simulink model "point_cloud_fusion_node"  (R2021b)
settings: Solver=FixedStepAuto  StartTime=0.0  StopTime=10.0  RelTol=1e-3
model workspace (MAT data in the model file):
  SL_ROS_VariableLengthArrays_MaxSizes.CommonInfo.ArrayTruncateAction = 'EmitWarning'
  SL_ROS_VariableLengthArrays_MaxSizes.MsgTypeMap = containers.Map
  SL_ROS_VariableLengthArrays_MaxSizes.MsgTypeMap.serialization.keys = {'sensor_msgs/PointCloud2'}
  SL_ROS_VariableLengthArrays_MaxSizes.MsgTypeMap.serialization.values{1}(1).PropertyName = 'data'
  SL_ROS_VariableLengthArrays_MaxSizes.MsgTypeMap.serialization.values{1}(1).DataType = 'uint8'
  SL_ROS_VariableLengthArrays_MaxSizes.MsgTypeMap.serialization.values{1}(1).MaxLength = 55000
  SL_ROS_VariableLengthArrays_MaxSizes.MsgTypeMap.serialization.values{1}(2).PropertyName = 'fields'
  SL_ROS_VariableLengthArrays_MaxSizes.MsgTypeMap.serialization.values{1}(2).DataType = 'sensor_msgs/PointField'
  SL_ROS_VariableLengthArrays_MaxSizes.MsgTypeMap.serialization.values{1}(2).MaxLength = 16
  SL_ROS_VariableLengthArrays_MaxSizes.MsgTypeMap.serialization.uniformity = 0
  SL_ROS_VariableLengthArrays_MaxSizes.MsgTypeMap.serialization.keyType = 'char'
  SL_ROS_VariableLengthArrays_MaxSizes.MsgTypeMap.serialization.valueType = 'any'
undefined symbols (not defined in the file): data, header, height, row_step, width
libraries: ros2lib x9, simulink x4
settings Model: Creator=takum  LastModifiedBy=takumi onozawa
settings SolverCC: AlgebraicLoopSolver=TrustRegion
settings OptimizationCC: EnhancedBackFolding=on  PassReuseOutputArgsAs=Individual arguments  ZeroExternalMemoryAtStartup=off  ZeroInternalMemoryAtStartup=off  MaxStackSize=64  OptimizeBlockOrder=speed  DifferentSizesBufferReuse=on  OptimizationCustomize=off  EfficientTunableParamExpr=on
settings DebuggingCC: ParameterTunabilityLossMsg=error  SFMachineParentedDataDiag=warning
settings SFSimCC: MATLABDynamicMemAlloc=off  SimTargetLang=C++
settings RTWCC: Description=Embedded Coder  SystemTargetFile=ert.tlc  HardwareBoard=Robot Operating System 2 (ROS 2)  GenCodeOnly=on  TemplateMakefile=ert_default_tmf  Toolchain=Colcon Tools  TargetLang=C++
settings CodeAppCC: ForceParamTrailComments=on  IgnoreCustomStorageClasses=off  OperatorAnnotations=on  SimulinkDataObjDesc=on  SFDataObjDesc=on  InsertBlockDesc=on
settings ERTTargetCC: CodeInterfacePackaging=C++ class  SupportVariableSizeSignals=on  RootIOFormat=Structure reference

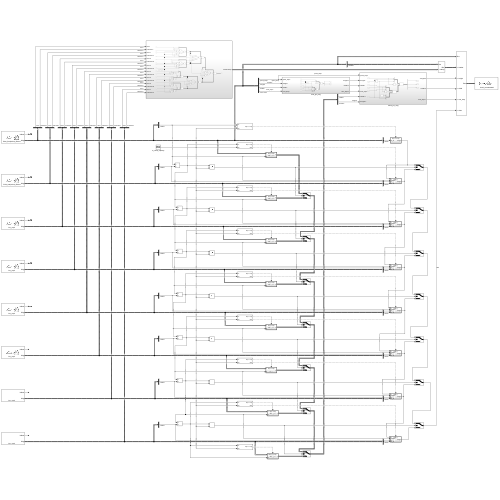
[thumbnail: Simulink's stored preview of the top-level diagram]
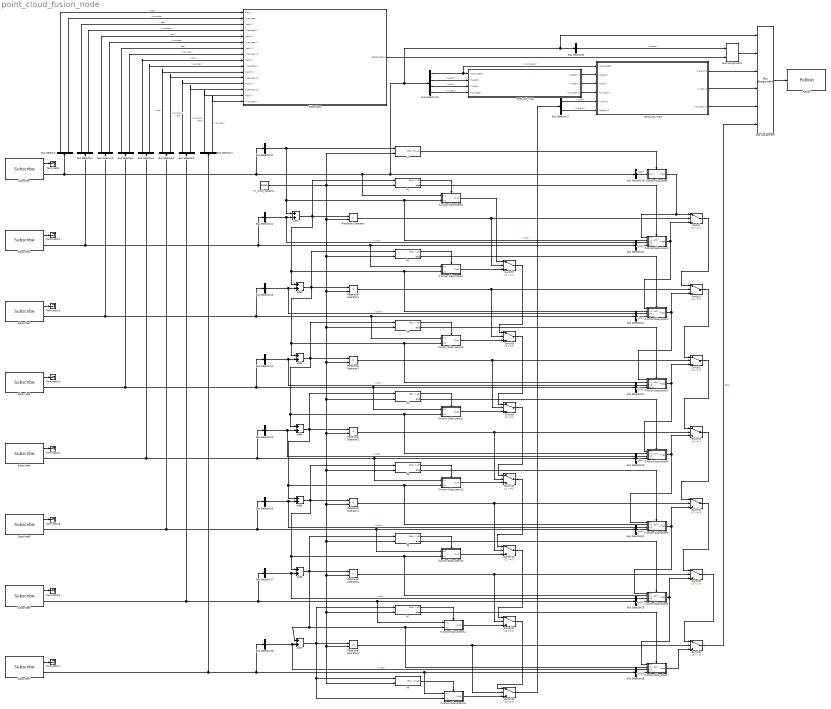
== system point_cloud_fusion_node ==
  Add{1..7} (7 alike) : Sum
  Bus Assignment : BusAssignment  AssignedSignals=header,height,width,row_step,data
  Bus Assignment1 : BusAssignment  AssignedSignals=stamp
  Bus Selector{,1..7} (8 alike) : BusSelector  OutputSignals=header.stamp.sec,header.stamp.nanosec
  Bus Selector10 : BusSelector  OutputSignals=point_step,height,width,row_step
  Bus Selector{11..18} (8 alike) : BusSelector  OutputSignals=width
  Bus Selector{19..26} (8 alike) : BusSelector  OutputSignals=data
  Bus Selector27 : BusSelector  OutputSignals=width,height
  Bus Selector8 : BusSelector  OutputSignals=header
  If : If  NumInputs=2  IfExpression=u1 <= u2  ShowElse=off
  If Action Subsystem : Subsystem  TreatAsAtomicUnit=on
  If Action Subsystem1 : Subsystem  TreatAsAtomicUnit=on
  If Action Subsystem10 : Subsystem  TreatAsAtomicUnit=on
  If Action Subsystem11 : Subsystem  TreatAsAtomicUnit=on
  If Action Subsystem12 : Subsystem  TreatAsAtomicUnit=on
  If Action Subsystem13 : Subsystem  TreatAsAtomicUnit=on
  If Action Subsystem14 : Subsystem  TreatAsAtomicUnit=on
  If Action Subsystem15 : Subsystem  TreatAsAtomicUnit=on
  If Action Subsystem2 : Subsystem  TreatAsAtomicUnit=on
  If Action Subsystem3 : Subsystem  TreatAsAtomicUnit=on
  If Action Subsystem4 : Subsystem  TreatAsAtomicUnit=on
  If Action Subsystem5 : Subsystem  TreatAsAtomicUnit=on
  If Action Subsystem6 : Subsystem  TreatAsAtomicUnit=on
  If Action Subsystem7 : Subsystem  TreatAsAtomicUnit=on
  If Action Subsystem8 : Subsystem  TreatAsAtomicUnit=on
  If Action Subsystem9 : Subsystem  TreatAsAtomicUnit=on
  If{1..7} (7 alike) : If  NumInputs=2  IfExpression=u1 > u2
  If8 : If  NumInputs=2  IfExpression=u1 <= u2  ShowElse=off
  Publish : ros2lib/Publish  topicSource=Specify your own  topic=cloud_concatenated  messageType=sensor_msgs/PointCloud2  QOSHistory=Keep last  QOSDepth=1  QOSReliability=Reliable  QOSDurability=Volatile
      settings: SourceProductBaseCode=RR
  Relational Operator{,1..6} (7 alike) : RelationalOperator  Operator=>  OutDataTypeStr=boolean  RndMeth=Simplest
  Subscribe : ros2lib/Subscribe  topicSource=Specify your own  topic=/lidar_front/points_filtered  messageType=sensor_msgs/PointCloud2  sampleTime=-1  QOSHistory=Keep last  QOSDepth=1  QOSReliability=Reliable  QOSDurability=Volatile
      settings: SourceProductBaseCode=RR
  Subscribe1 : ros2lib/Subscribe  topicSource=Specify your own  topic=/lidar_rear/points_filtered  messageType=sensor_msgs/PointCloud2  sampleTime=-1  QOSHistory=Keep last  QOSDepth=1  QOSReliability=Reliable  QOSDurability=Volatile
      settings: SourceProductBaseCode=RR
  Subscribe{2..7} (6 alike) : ros2lib/Subscribe  topicSource=Specify your own  topic=/my_topic  messageType=sensor_msgs/PointCloud2  sampleTime=-1  QOSHistory=Keep last  QOSDepth=1  QOSReliability=Reliable  QOSDurability=Volatile
      settings: SourceProductBaseCode=RR
  Subsystem : Subsystem
  Switch{,1..13} (14 alike) : Switch  Criteria=u2 ~= 0
  Terminator{,1..7} (8 alike) : Terminator
  m_cloud_capacity : Constant  Value=55000  OutDataTypeStr=uint32
  reset_pcl_msg : Subsystem
  resize_pcl_msg : Subsystem
  wires:
  Bus Selector10/1 -> resize_pcl_msg/1(<point_step>), reset_pcl_msg/1(<point_step>)  "<point_step>"
  If Action Subsystem7/1(msgs) -> Switch6/3
  If Action Subsystem2/1(msgs) -> Switch1/3, If Action Subsystem3/1(In1)
  Bus Selector19/1 -> If Action Subsystem/1(pc_in)  "<data>"
  Subscribe2/2 -> Bus Selector2/1, Bus Selector13/1, If Action Subsystem10/1(In1), Bus Selector21/1
  If5/1 -> If Action Subsystem12/Action
  Relational Operator6/1 -> Switch13/2, Switch6/2
  If7/2 -> If Action Subsystem7/Action
  Switch10/1 -> Switch11/1
  Subscribe1/1 -> Terminator1/1
  If Action Subsystem12/1(Out1) -> Switch10/3
  Bus Selector21/1 -> If Action Subsystem2/4(pc_in)  "<data>"
  Switch9/1 -> Switch10/1
  If Action Subsystem11/1(Out1) -> Switch9/3
  If3/1 -> If Action Subsystem10/Action
  Bus Selector24/1 -> If Action Subsystem5/4(pc_in)  "<data>"
  Bus Selector23/1 -> If Action Subsystem4/4(pc_in)  "<data>"
  Switch4/1 -> Switch5/1
  Subscribe/2 -> Bus Selector/1, Bus Selector11/1, If Action Subsystem8/1(In1), Bus Selector19/1, Bus Selector8/1, Bus Assignment/1, Bus Selector10/1
  Switch2/1 -> Switch3/1
  If1/1 -> If Action Subsystem8/Action
  If Action Subsystem3/1(msgs) -> Switch2/3, If Action Subsystem4/1(In1)
  If6/2 -> If Action Subsystem6/Action
  Bus Assignment/1 -> Publish/1
  Bus Selector14/1 -> Add3/2, If Action Subsystem3/3(In3)  "<width>"
  If4/2 -> If Action Subsystem4/Action
  If2/2 -> If Action Subsystem2/Action
  Subscribe5/2 -> Bus Selector5/1, If Action Subsystem13/1(In1), Bus Selector24/1, Bus Selector16/1
  If3/2 -> If Action Subsystem3/Action
  Add1/1 -> Relational Operator/1, If1/1, Add2/1, If Action Subsystem9/2(In2), If Action Subsystem2/2(<width>)
  If Action Subsystem/1(msgs) -> Switch/1, If Action Subsystem1/1(In1)
  Bus Assignment1/1 -> Bus Assignment/2
  Switch3/1 -> Switch4/1
  Switch/1 -> Switch1/1
  Switch12/1 -> Switch13/1
  Add3/1 -> If Action Subsystem11/2(In2), If Action Subsystem4/2(<width>), Add4/1, If3/1, Relational Operator2/1
  Subscribe/1 -> Terminator/1
  Add2/1 -> If2/1, Add3/1, If Action Subsystem10/2(In2), If Action Subsystem3/2(<width>), Relational Operator1/1
  Relational Operator2/1 -> Switch2/2, Switch9/2
  Bus Selector18/1 -> If Action Subsystem7/3(In3), Add7/2  "<width>"
  Bus Selector25/1 -> If Action Subsystem6/4(pc_in)  "<data>"
  If Action Subsystem15/1(Out1) -> Switch13/3
  If Action Subsystem13/1(Out1) -> Switch11/3
  Subscribe6/2 -> Bus Selector6/1, Bus Selector25/1, If Action Subsystem14/1(In1), Bus Selector17/1
  Bus Selector17/1 -> Add6/2, If Action Subsystem6/3(In3)  "<width>"
  Relational Operator3/1 -> Switch3/2, Switch10/2
  If1/2 -> If Action Subsystem1/Action
  If2/1 -> If Action Subsystem9/Action
  If Action Subsystem8/1(Out1) -> Switch7/1
  If7/1 -> If Action Subsystem14/Action
  Bus Selector12/1 -> Add1/2, If Action Subsystem1/3(In3)  "<width>"
  Relational Operator5/1 -> Switch12/2, Switch5/2
  If Action Subsystem4/1(msgs) -> Switch3/3, If Action Subsystem5/1(In1)
  If Action Subsystem10/1(Out1) -> Switch8/3
  Add6/1 -> If Action Subsystem14/2(In2), If Action Subsystem7/2(<width>), Add7/1, If6/1, Relational Operator5/1
  Switch6/1 -> Bus Assignment/6  "data"
  Add5/1 -> If Action Subsystem13/2(In2), If Action Subsystem6/2(<width>), Add6/1, If5/1, Relational Operator4/1
  If8/1 -> If Action Subsystem15/Action
  If5/2 -> If Action Subsystem5/Action
  Switch5/1 -> Switch6/1
  Switch1/1 -> Switch2/1
  Subscribe3/2 -> Bus Selector3/1, Bus Selector14/1, If Action Subsystem11/1(In1), Bus Selector22/1
  Bus Selector20/1 -> If Action Subsystem1/4(pc_in)  "<data>"
  If Action Subsystem5/1(msgs) -> Switch4/3, If Action Subsystem6/1(In1)
  Bus Selector15/1 -> Add4/2, If Action Subsystem4/3(In3)  "<width>"
  Switch8/1 -> Switch9/1
  If/1 -> If Action Subsystem/Action
  Relational Operator4/1 -> Switch4/2, Switch11/2
  If Action Subsystem6/1(msgs) -> Switch5/3, If Action Subsystem7/1(In1)
  Switch7/1 -> Switch8/1
  Bus Selector8/1 -> Bus Assignment1/1  "<header>"
  m_cloud_capacity/1 -> If3/2, Relational Operator2/2, Relational Operator3/2, Relational Operator4/2, If7/2, If8/2, Relational Operator6/2, Relational Operator5/2, If6/2, If5/2, If4/2, Relational Operator1/2, If2/2, Relational Operator/2, If/2, If1/2
  Bus Selector22/1 -> If Action Subsystem3/4(pc_in)  "<data>"
  Bus Selector11/1 -> If Action Subsystem8/2(In2), If Action Subsystem1/2(<width>), Add1/1, If/1  "<width>"
  Bus Selector26/1 -> If Action Subsystem7/4(pc_in)  "<data>"
  Add7/1 -> If8/1, If Action Subsystem15/2(In2), If7/1, Relational Operator6/1
  Bus Selector16/1 -> Add5/2, If Action Subsystem5/3(In3)  "<width>"
  If6/1 -> If Action Subsystem13/Action
  If Action Subsystem14/1(Out1) -> Switch12/3
  Relational Operator1/1 -> Switch1/2, Switch8/2
  Switch13/1 -> Bus Selector27/1
  Relational Operator/1 -> Switch/2, Switch7/2
  Subscribe4/2 -> Bus Selector4/1, Bus Selector15/1, Bus Selector23/1, If Action Subsystem12/1(In1)
  Switch11/1 -> Switch12/1
  Bus Selector13/1 -> Add2/2, If Action Subsystem2/3(In3)  "<width>"
  Add4/1 -> If4/1, If Action Subsystem12/2(In2), If Action Subsystem5/2(<width>), Add5/1, Relational Operator3/1
  If Action Subsystem1/1(msgs) -> Switch/3, If Action Subsystem2/1(In1)
  Subscribe1/2 -> Bus Selector1/1, Bus Selector12/1, If Action Subsystem9/1(In1), Bus Selector20/1
  Subscribe7/2 -> Bus Selector7/1, Bus Selector18/1, If Action Subsystem15/1(In1), Bus Selector26/1
  If Action Subsystem9/1(Out1) -> Switch7/3
  If4/1 -> If Action Subsystem11/Action
  Subscribe2/1 -> Terminator2/1
  Subscribe3/1 -> Terminator3/1
  Subscribe4/1 -> Terminator4/1
  Subscribe5/1 -> Terminator5/1
  Subscribe6/1 -> Terminator6/1
  Subscribe7/1 -> Terminator7/1
  Bus Selector27/1 -> resize_pcl_msg/5(<width>1)  "<width>"
  Bus Selector27/2 -> resize_pcl_msg/6(<height>1)  "<height>"
  resize_pcl_msg/1(<height>2) -> Bus Assignment/3
  resize_pcl_msg/2(<width>2) -> Bus Assignment/4
  resize_pcl_msg/3(<row_step>1) -> Bus Assignment/5
  Bus Selector10/2 -> reset_pcl_msg/2(<height>)  "<height>"
  Bus Selector10/3 -> reset_pcl_msg/3(<width>)  "<width>"
  Bus Selector10/4 -> reset_pcl_msg/4(<row_step>)  "<row_step>"
  reset_pcl_msg/1(<height>1) -> resize_pcl_msg/2(<height>)
  reset_pcl_msg/2(<width>1) -> resize_pcl_msg/3(<width>)
  reset_pcl_msg/3(<row_step>1) -> resize_pcl_msg/4(<row_step>)
  Bus Selector/1 -> Subsystem/1(<sec>)  "<sec>"
  Bus Selector/2 -> Subsystem/2(<nanosec>)  "<nanosec>"
  Bus Selector1/1 -> Subsystem/3(<sec>1)  "<sec>"
  Bus Selector1/2 -> Subsystem/4(<nanosec>1)  "<nanosec>"
  Bus Selector2/1 -> Subsystem/5(<sec>2)  "<sec>"
  Bus Selector2/2 -> Subsystem/6(<nanosec>2)  "<nanosec>"
  Bus Selector3/1 -> Subsystem/7(<sec>3)  "<sec>"
  Bus Selector3/2 -> Subsystem/8(<nanosec>3)  "<nanosec>"
  Bus Selector4/1 -> Subsystem/9(<sec>4)  "<sec>"
  Bus Selector4/2 -> Subsystem/10(<nanosec>4)  "<nanosec>"
  Bus Selector5/1 -> Subsystem/11(<sec>5)  "<sec>"
  Bus Selector5/2 -> Subsystem/12(<nanosec>5)  "<nanosec>"
  Bus Selector6/1 -> Subsystem/13(<sec>6)  "<sec>"
  Bus Selector6/2 -> Subsystem/14(<nanosec>6)  "<nanosec>"
  Bus Selector7/1 -> Subsystem/15(<sec>7)  "<sec>"
  Bus Selector7/2 -> Subsystem/16(<nanosec>7)  "<nanosec>"
  Subsystem/1(header.stamp) -> Bus Assignment1/2

== system point_cloud_fusion_node/If Action Subsystem ==
  pc_in : Inport
  Action Port : ActionPort  ActionPortLabel=if(u1 <= u2)
  msgs : Outport
  wires:
  pc_in/1 -> msgs/1

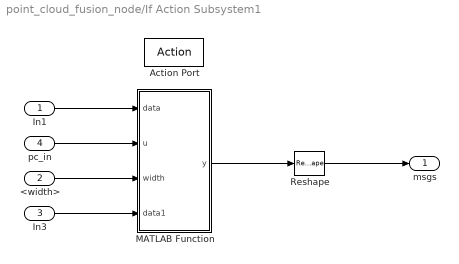
== system point_cloud_fusion_node/If Action Subsystem1 ==
  In1 : Inport
  <width> : Inport  Port=2
  In3 : Inport  Port=3
  pc_in : Inport  Port=4
  Action Port : ActionPort  ActionPortLabel=else
  MATLAB Function : MATLAB Function  TreatAsAtomicUnit=on
  Reshape : Reshape
  msgs : Outport
  wires:
  pc_in/1 -> MATLAB Function/2(u)
  MATLAB Function/1(y) -> Reshape/1
  In1/1 -> MATLAB Function/1(data)
  <width>/1 -> MATLAB Function/3(width)
  In3/1 -> MATLAB Function/4(data1)
  Reshape/1 -> msgs/1

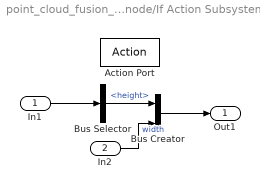
== system point_cloud_fusion_node/If Action Subsystem10 ==
  In1 : Inport
  In2 : Inport  Port=2
  Action Port : ActionPort  ActionPortLabel=if(u1 > u2)
  Bus Creator : BusCreator  Inputs=2
  Bus Selector : BusSelector  OutputSignals=height
  Out1 : Outport
  wires:
  In1/1 -> Bus Selector/1
  Bus Selector/1 -> Bus Creator/1  "<height>"
  Bus Creator/1 -> Out1/1
  In2/1 -> Bus Creator/2  "width"

== system point_cloud_fusion_node/If Action Subsystem11 ==
  In1 : Inport
  In2 : Inport  Port=2
  Action Port : ActionPort  ActionPortLabel=if(u1 > u2)
  Bus Creator : BusCreator  Inputs=2
  Bus Selector : BusSelector  OutputSignals=height
  Out1 : Outport
  wires:
  In1/1 -> Bus Selector/1
  Bus Selector/1 -> Bus Creator/1  "<height>"
  Bus Creator/1 -> Out1/1
  In2/1 -> Bus Creator/2  "width"

== system point_cloud_fusion_node/If Action Subsystem12 ==
  In1 : Inport
  In2 : Inport  Port=2
  Action Port : ActionPort  ActionPortLabel=if(u1 > u2)
  Bus Creator : BusCreator  Inputs=2
  Bus Selector : BusSelector  OutputSignals=height
  Out1 : Outport
  wires:
  In1/1 -> Bus Selector/1
  Bus Selector/1 -> Bus Creator/1  "<height>"
  Bus Creator/1 -> Out1/1
  In2/1 -> Bus Creator/2  "width"

== system point_cloud_fusion_node/If Action Subsystem13 ==
  In1 : Inport
  In2 : Inport  Port=2
  Action Port : ActionPort  ActionPortLabel=if(u1 > u2)
  Bus Creator1 : BusCreator  Inputs=2
  Bus Selector1 : BusSelector  OutputSignals=height
  Out1 : Outport
  wires:
  Bus Creator1/1 -> Out1/1
  In2/1 -> Bus Creator1/2  "width"
  Bus Selector1/1 -> Bus Creator1/1  "<height>"
  In1/1 -> Bus Selector1/1

== system point_cloud_fusion_node/If Action Subsystem14 ==
  In1 : Inport
  In2 : Inport  Port=2
  Action Port : ActionPort  ActionPortLabel=if(u1 > u2)
  Bus Creator : BusCreator  Inputs=2
  Bus Selector : BusSelector  OutputSignals=height
  Out1 : Outport
  wires:
  In1/1 -> Bus Selector/1
  Bus Selector/1 -> Bus Creator/1  "<height>"
  Bus Creator/1 -> Out1/1
  In2/1 -> Bus Creator/2  "width"

== system point_cloud_fusion_node/If Action Subsystem15 ==
  In1 : Inport
  In2 : Inport  Port=2
  Action Port : ActionPort  ActionPortLabel=if(u1 <= u2)
  Bus Creator : BusCreator  Inputs=2
  Bus Selector : BusSelector  OutputSignals=height
  Out1 : Outport
  wires:
  In1/1 -> Bus Selector/1
  Bus Selector/1 -> Bus Creator/1  "<height>"
  Bus Creator/1 -> Out1/1
  In2/1 -> Bus Creator/2  "width"

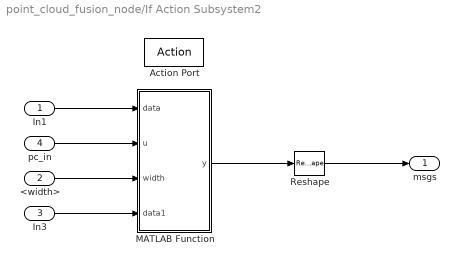
== system point_cloud_fusion_node/If Action Subsystem2 ==
  In1 : Inport
  <width> : Inport  Port=2
  In3 : Inport  Port=3
  pc_in : Inport  Port=4
  Action Port : ActionPort  ActionPortLabel=else
  MATLAB Function : MATLAB Function  TreatAsAtomicUnit=on
  Reshape : Reshape
  msgs : Outport
  wires:
  pc_in/1 -> MATLAB Function/2(u)
  MATLAB Function/1(y) -> Reshape/1
  In1/1 -> MATLAB Function/1(data)
  <width>/1 -> MATLAB Function/3(width)
  In3/1 -> MATLAB Function/4(data1)
  Reshape/1 -> msgs/1

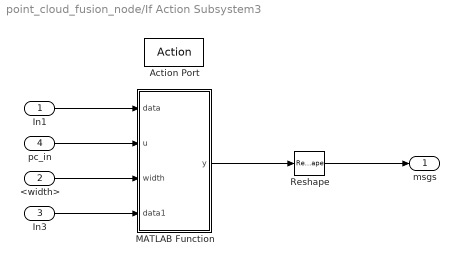
== system point_cloud_fusion_node/If Action Subsystem3 ==
  In1 : Inport
  <width> : Inport  Port=2
  In3 : Inport  Port=3
  pc_in : Inport  Port=4
  Action Port : ActionPort  ActionPortLabel=else
  MATLAB Function : MATLAB Function  TreatAsAtomicUnit=on
  Reshape : Reshape
  msgs : Outport
  wires:
  pc_in/1 -> MATLAB Function/2(u)
  MATLAB Function/1(y) -> Reshape/1
  In1/1 -> MATLAB Function/1(data)
  <width>/1 -> MATLAB Function/3(width)
  In3/1 -> MATLAB Function/4(data1)
  Reshape/1 -> msgs/1

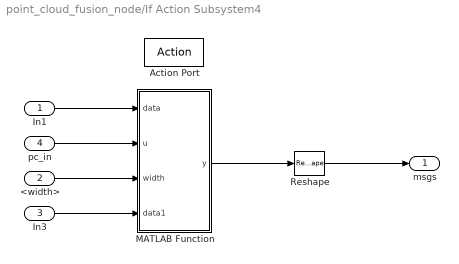
== system point_cloud_fusion_node/If Action Subsystem4 ==
  In1 : Inport
  <width> : Inport  Port=2
  In3 : Inport  Port=3
  pc_in : Inport  Port=4
  Action Port : ActionPort  ActionPortLabel=else
  MATLAB Function : MATLAB Function  TreatAsAtomicUnit=on
  Reshape : Reshape
  msgs : Outport
  wires:
  pc_in/1 -> MATLAB Function/2(u)
  MATLAB Function/1(y) -> Reshape/1
  In1/1 -> MATLAB Function/1(data)
  <width>/1 -> MATLAB Function/3(width)
  In3/1 -> MATLAB Function/4(data1)
  Reshape/1 -> msgs/1

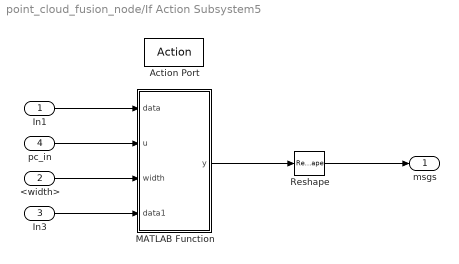
== system point_cloud_fusion_node/If Action Subsystem5 ==
  In1 : Inport
  <width> : Inport  Port=2
  In3 : Inport  Port=3
  pc_in : Inport  Port=4
  Action Port : ActionPort  ActionPortLabel=else
  MATLAB Function : MATLAB Function  TreatAsAtomicUnit=on
  Reshape : Reshape
  msgs : Outport
  wires:
  pc_in/1 -> MATLAB Function/2(u)
  MATLAB Function/1(y) -> Reshape/1
  In1/1 -> MATLAB Function/1(data)
  <width>/1 -> MATLAB Function/3(width)
  In3/1 -> MATLAB Function/4(data1)
  Reshape/1 -> msgs/1

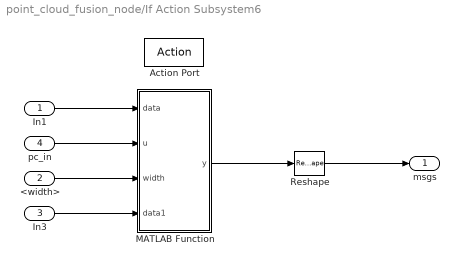
== system point_cloud_fusion_node/If Action Subsystem6 ==
  In1 : Inport
  <width> : Inport  Port=2
  In3 : Inport  Port=3
  pc_in : Inport  Port=4
  Action Port : ActionPort  ActionPortLabel=else
  MATLAB Function : MATLAB Function  TreatAsAtomicUnit=on
  Reshape : Reshape
  msgs : Outport
  wires:
  pc_in/1 -> MATLAB Function/2(u)
  MATLAB Function/1(y) -> Reshape/1
  In1/1 -> MATLAB Function/1(data)
  <width>/1 -> MATLAB Function/3(width)
  In3/1 -> MATLAB Function/4(data1)
  Reshape/1 -> msgs/1

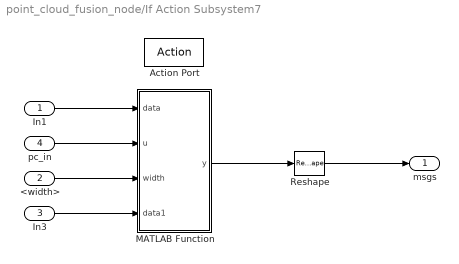
== system point_cloud_fusion_node/If Action Subsystem7 ==
  In1 : Inport
  <width> : Inport  Port=2
  In3 : Inport  Port=3
  pc_in : Inport  Port=4
  Action Port : ActionPort  ActionPortLabel=else
  MATLAB Function : MATLAB Function  TreatAsAtomicUnit=on
  Reshape : Reshape
  msgs : Outport
  wires:
  pc_in/1 -> MATLAB Function/2(u)
  MATLAB Function/1(y) -> Reshape/1
  In1/1 -> MATLAB Function/1(data)
  <width>/1 -> MATLAB Function/3(width)
  In3/1 -> MATLAB Function/4(data1)
  Reshape/1 -> msgs/1

== system point_cloud_fusion_node/If Action Subsystem8 ==
  In1 : Inport
  In2 : Inport  Port=2
  Action Port : ActionPort  ActionPortLabel=if(u1 > u2)
  Bus Creator : BusCreator  Inputs=2
  Bus Selector : BusSelector  OutputSignals=height
  Out1 : Outport
  wires:
  In1/1 -> Bus Selector/1
  Bus Selector/1 -> Bus Creator/1  "<height>"
  Bus Creator/1 -> Out1/1
  In2/1 -> Bus Creator/2  "width"

== system point_cloud_fusion_node/If Action Subsystem9 ==
  In1 : Inport
  In2 : Inport  Port=2
  Action Port : ActionPort  ActionPortLabel=if(u1 > u2)
  Bus Creator : BusCreator  Inputs=2
  Bus Selector : BusSelector  OutputSignals=height
  Out1 : Outport
  wires:
  In1/1 -> Bus Selector/1
  Bus Selector/1 -> Bus Creator/1  "<height>"
  Bus Creator/1 -> Out1/1
  In2/1 -> Bus Creator/2  "width"

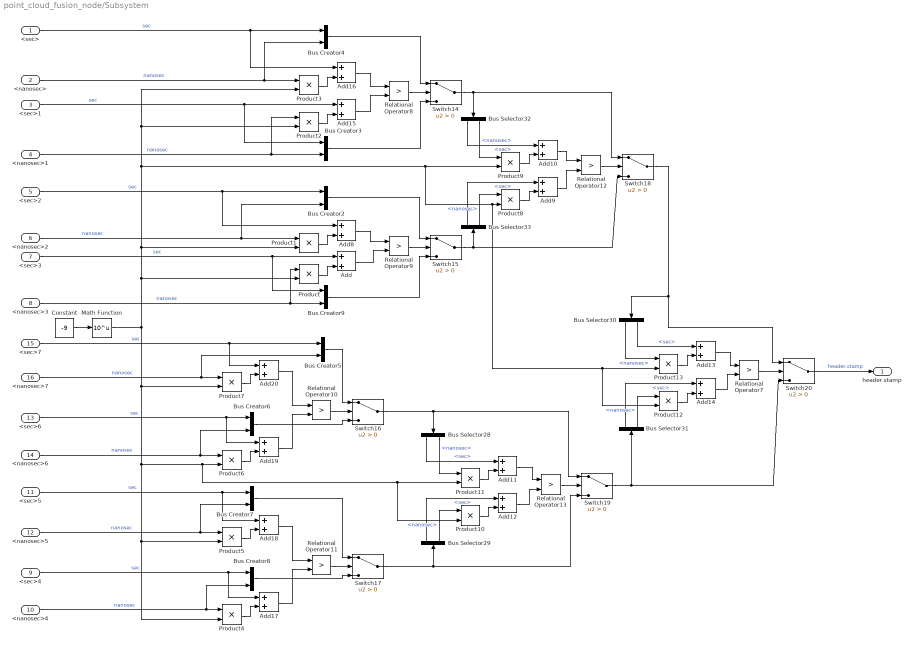
== system point_cloud_fusion_node/Subsystem ==
  <sec> : Inport
  <nanosec> : Inport  Port=2
  <sec>1 : Inport  Port=3
  <nanosec>1 : Inport  Port=4
  <sec>2 : Inport  Port=5
  <nanosec>2 : Inport  Port=6
  <sec>3 : Inport  Port=7
  <nanosec>3 : Inport  Port=8
  <sec>4 : Inport  Port=9
  <nanosec>4 : Inport  Port=10
  <sec>5 : Inport  Port=11
  <nanosec>5 : Inport  Port=12
  <sec>6 : Inport  Port=13
  <nanosec>6 : Inport  Port=14
  <sec>7 : Inport  Port=15
  <nanosec>7 : Inport  Port=16
  Add{,8..20} (14 alike) : Sum
  Bus Creator{2..9} (8 alike) : BusCreator  Inputs=2
  Bus Selector{28..29,31..33} (5 alike) : BusSelector  OutputSignals=sec,nanosec
  Bus Selector30 : BusSelector  OutputSignals=nanosec,sec
  Constant : Constant  Value=-9
  Math Function : Math  Operator=10^u  SaturateOnIntegerOverflow=on
  Product{,1..13} (14 alike) : Product
  Relational Operator{7..13} (7 alike) : RelationalOperator  Operator=>  OutDataTypeStr=boolean  RndMeth=Simplest
  Switch{14..20} (7 alike) : Switch  Criteria=u2 > Threshold
  header.stamp : Outport
  wires:
  Add15/1 -> Relational Operator8/2
  <sec>6/1 -> Add19/1, Bus Creator6/1  "sec"
  <sec>/1 -> Add16/1, Bus Creator4/1  "sec"
  Bus Creator6/1 -> Switch16/3
  <nanosec>1/1 -> Product2/1, Bus Creator3/2  "nanosec"
  Bus Selector31/1 -> Add14/1  "<sec>"
  <nanosec>2/1 -> Bus Creator2/2, Product1/1  "nanosec"
  Relational Operator13/1 -> Switch19/2
  Add14/1 -> Relational Operator7/2
  <sec>2/1 -> Add8/1, Bus Creator2/1  "sec"
  Add20/1 -> Relational Operator10/1
  Bus Selector29/2 -> Product10/1  "<nanosec>"
  Bus Creator9/1 -> Switch15/3
  Relational Operator7/1 -> Switch20/2
  Bus Creator7/1 -> Switch17/1
  Bus Creator4/1 -> Switch14/1
  <sec>4/1 -> Bus Creator8/1, Add17/1  "sec"
  Product4/1 -> Add17/2
  Bus Creator3/1 -> Switch14/3
  <nanosec>4/1 -> Bus Creator8/2, Product4/1  "nanosec"
  Switch17/1 -> Switch19/3, Bus Selector29/1
  Add10/1 -> Relational Operator12/1
  <nanosec>5/1 -> Bus Creator7/2, Product5/1  "nanosec"
  <sec>7/1 -> Add20/1, Bus Creator5/1  "sec"
  Constant/1 -> Math Function/1
  Product2/1 -> Add15/2
  Bus Selector30/1 -> Product13/1  "<nanosec>"
  Switch16/1 -> Switch19/1, Bus Selector28/1
  Bus Creator8/1 -> Switch17/3
  <nanosec>6/1 -> Bus Creator6/2, Product6/1  "nanosec"
  Bus Creator2/1 -> Switch15/1
  Product1/1 -> Add8/2
  <sec>3/1 -> Bus Creator9/1, Add/1  "sec"
  Relational Operator10/1 -> Switch16/2
  Relational Operator9/1 -> Switch15/2
  Add16/1 -> Relational Operator8/1
  Switch18/1 -> Bus Selector30/1, Switch20/1
  Bus Selector31/2 -> Product12/1  "<nanosec>"
  Switch15/1 -> Bus Selector33/1, Switch18/3
  <nanosec>7/1 -> Bus Creator5/2, Product7/1  "nanosec"
  Math Function/1 -> Product4/2, Product5/2, Product10/2, Product11/2, Product6/2, Product7/2, Product2/2, Product3/2, Product13/2, Product12/2, Product8/2, Product9/2, Product1/2, Product/2
  Switch19/1 -> Bus Selector31/1, Switch20/3
  Product5/1 -> Add18/2
  Bus Creator5/1 -> Switch16/1
  Add17/1 -> Relational Operator11/2
  Bus Selector32/2 -> Product9/1  "<nanosec>"
  Product7/1 -> Add20/2
  Bus Selector28/1 -> Add11/1  "<sec>"
  Bus Selector33/1 -> Add9/1  "<sec>"
  Add8/1 -> Relational Operator9/1
  <sec>5/1 -> Add18/1, Bus Creator7/1  "sec"
  Product8/1 -> Add9/2
  Product6/1 -> Add19/2
  Switch14/1 -> Switch18/1, Bus Selector32/1
  Product13/1 -> Add13/2
  Add12/1 -> Relational Operator13/2
  Add13/1 -> Relational Operator7/1
  Product/1 -> Add/2
  Bus Selector30/2 -> Add13/1  "<sec>"
  Add11/1 -> Relational Operator13/1
  <nanosec>/1 -> Product3/1, Bus Creator4/2  "nanosec"
  Bus Selector32/1 -> Add10/1  "<sec>"
  Product12/1 -> Add14/2
  Product11/1 -> Add11/2
  Product3/1 -> Add16/2
  Product10/1 -> Add12/2
  <nanosec>3/1 -> Bus Creator9/2, Product/1  "nanosec"
  Add9/1 -> Relational Operator12/2
  Relational Operator11/1 -> Switch17/2
  Add/1 -> Relational Operator9/2
  Add19/1 -> Relational Operator10/2
  Bus Selector33/2 -> Product8/1  "<nanosec>"
  <sec>1/1 -> Bus Creator3/1, Add15/1  "sec"
  Product9/1 -> Add10/2
  Add18/1 -> Relational Operator11/1
  Relational Operator12/1 -> Switch18/2
  Bus Selector29/1 -> Add12/1  "<sec>"
  Bus Selector28/2 -> Product11/1  "<nanosec>"
  Relational Operator8/1 -> Switch14/2
  Switch20/1 -> header.stamp/1  "header.stamp"

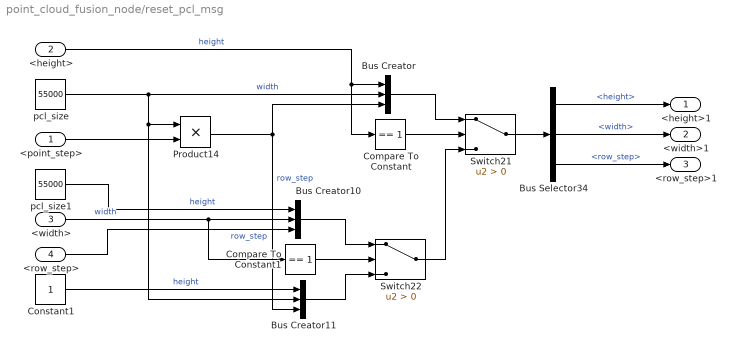
== system point_cloud_fusion_node/reset_pcl_msg ==
  <point_step> : Inport
  <height> : Inport  Port=2
  <width> : Inport  Port=3
  <row_step> : Inport  Port=4
  Bus Creator : BusCreator  Inputs=3
  Bus Creator10 : BusCreator  Inputs=3
  Bus Creator11 : BusCreator  Inputs=3
  Bus Selector34 : BusSelector  OutputSignals=height,width,row_step
  Compare To Constant : simulink/Logic and Bit Operations/Compare To Constant  relop===  const=1  OutDataTypeStr=boolean
  Compare To Constant1 : simulink/Logic and Bit Operations/Compare To Constant  relop===  const=1  OutDataTypeStr=boolean
  Constant1 : Constant
  Product14 : Product
  Switch21 : Switch  Criteria=u2 > Threshold
  Switch22 : Switch  Criteria=u2 > Threshold
  pcl_size : Constant  Value=55000
  pcl_size1 : Constant  Value=55000
  <height>1 : Outport
  <width>1 : Outport  Port=2
  <row_step>1 : Outport  Port=3
  wires:
  <width>/1 -> Compare To Constant1/1, Bus Creator10/2  "width"
  <height>/1 -> Compare To Constant/1, Bus Creator/1  "height"
  Bus Creator11/1 -> Switch22/3
  Switch21/1 -> Bus Selector34/1
  Switch22/1 -> Switch21/3
  Compare To Constant1/1 -> Switch22/2
  Compare To Constant/1 -> Switch21/2
  Bus Selector34/2 -> <width>1/1  "<width>"
  Bus Creator10/1 -> Switch22/1
  pcl_size/1 -> Bus Creator/2, Product14/1, Bus Creator11/2  "width"
  Constant1/1 -> Bus Creator11/1  "height"
  pcl_size1/1 -> Bus Creator10/1  "height"
  Product14/1 -> Bus Creator/3, Bus Creator11/3  "row_step"
  Bus Selector34/3 -> <row_step>1/1  "<row_step>"
  Bus Selector34/1 -> <height>1/1  "<height>"
  Bus Creator/1 -> Switch21/1
  <point_step>/1 -> Product14/2
  <row_step>/1 -> Bus Creator10/3  "row_step"

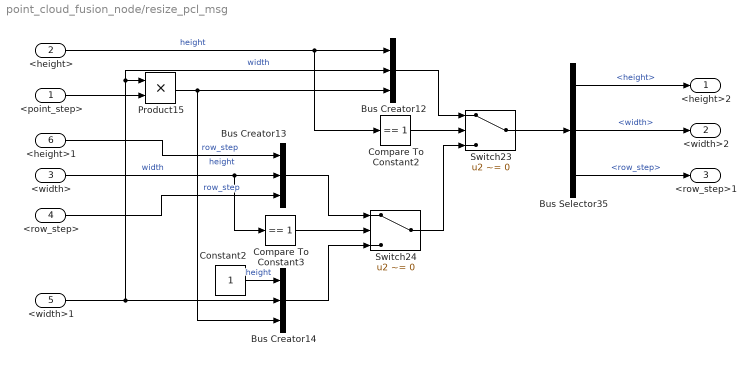
== system point_cloud_fusion_node/resize_pcl_msg ==
  <point_step> : Inport
  <height> : Inport  Port=2
  <width> : Inport  Port=3
  <row_step> : Inport  Port=4
  <width>1 : Inport  Port=5
  <height>1 : Inport  Port=6
  Bus Creator12 : BusCreator  Inputs=3
  Bus Creator13 : BusCreator  Inputs=3
  Bus Creator14 : BusCreator  Inputs=3
  Bus Selector35 : BusSelector  OutputSignals=height,width,row_step
  Compare To Constant2 : simulink/Logic and Bit Operations/Compare To Constant  relop===  const=1  OutDataTypeStr=boolean
  Compare To Constant3 : simulink/Logic and Bit Operations/Compare To Constant  relop===  const=1  OutDataTypeStr=boolean
  Constant2 : Constant
  Product15 : Product
  Switch23 : Switch  Criteria=u2 ~= 0
  Switch24 : Switch  Criteria=u2 ~= 0
  <height>2 : Outport
  <width>2 : Outport  Port=2
  <row_step>1 : Outport  Port=3
  wires:
  Bus Creator13/1 -> Switch24/1
  Constant2/1 -> Bus Creator14/1  "height"
  Bus Creator14/1 -> Switch24/3
  Bus Selector35/1 -> <height>2/1  "<height>"
  <width>1/1 -> Bus Creator14/2, Bus Creator12/2, Product15/1  "width"
  Bus Creator12/1 -> Switch23/1
  Switch23/1 -> Bus Selector35/1
  Bus Selector35/3 -> <row_step>1/1  "<row_step>"
  Product15/1 -> Bus Creator12/3, Bus Creator14/3  "row_step"
  Switch24/1 -> Switch23/3
  <height>1/1 -> Bus Creator13/1  "height"
  Compare To Constant2/1 -> Switch23/2
  Compare To Constant3/1 -> Switch24/2
  <width>/1 -> Compare To Constant3/1, Bus Creator13/2  "width"
  <height>/1 -> Compare To Constant2/1, Bus Creator12/1  "height"
  <row_step>/1 -> Bus Creator13/3  "row_step"
  Bus Selector35/2 -> <width>2/1  "<width>"
  <point_step>/1 -> Product15/2

== matlab function point_cloud_fusion_node/If Action Subsystem2/MATLAB Function ==
  data: data input; u input; y output; width input; data1 input
function y = fcn(data, u, width, data1)
s=width+1;
f=width+data1;
data(s:f)=u(1:data1);
y=data;

== matlab function point_cloud_fusion_node/If Action Subsystem1/MATLAB Function ==
  data: data input; u input; y output; width input; data1 input
function y = fcn(data, u, width, data1)
s=width+1;
f=width+data1;
data(s:f)=u(1:data1);
y=data;

== matlab function point_cloud_fusion_node/If Action Subsystem3/MATLAB Function ==
  data: data input; u input; y output; width input; data1 input
function y = fcn(data, u, width, data1)
s=width+1;
f=width+data1;
data(s:f)=u(1:data1);
y=data;

== matlab function point_cloud_fusion_node/If Action Subsystem4/MATLAB Function ==
  data: data input; u input; y output; width input; data1 input
function y = fcn(data, u, width, data1)
s=width+1;
f=width+data1;
data(s:f)=u(1:data1);
y=data;

== matlab function point_cloud_fusion_node/If Action Subsystem5/MATLAB Function ==
  data: data input; u input; y output; width input; data1 input
function y = fcn(data, u, width, data1)
s=width+1;
f=width+data1;
data(s:f)=u(1:data1);
y=data;

== matlab function point_cloud_fusion_node/If Action Subsystem6/MATLAB Function ==
  data: data input; u input; y output; width input; data1 input
function y = fcn(data, u, width, data1)
s=width+1;
f=width+data1;
data(s:f)=u(1:data1);
y=data;

== matlab function point_cloud_fusion_node/If Action Subsystem7/MATLAB Function ==
  data: data input; u input; y output; width input; data1 input
function y = fcn(data, u, width, data1)
s=width+1;
f=width+data1;
data(s:f)=u(1:data1);
y=data;
